simulink library "dkc"  (R2021b)
settings: Solver=VariableStepAuto  StartTime=0.0  StopTime=10.0  RelTol=1e-3
undefined symbols (not defined in the file or in its folder): ENUM_ANTITHEFT_ALARM, ENUM_ANTITHEFT_ARM, ENUM_ANTITHEFT_DISARM, ENUM_ANTITHEFT_WAIT, ENUM_BTCONNSTA_CONNECTED, ENUM_BTConnSta_CONNECTED, ENUM_BTCONNSTA_DISCONNECTED, ENUM_DKCAuthSta_DECRYPTIONFAIL, ENUM_DKCAuthSta_NORMAL, ENUM_DKCAuthSta_TIMEERROR, ENUM_DKCPCMDHANDING_FORCELIFT, ENUM_DKCPCMDHANDING_LOCK, ENUM_DKCPCMDHANDING_LOCKTGATEFAIL, ENUM_DKCPCMDHANDING_OVER, ENUM_DKCPCMDHANDING_TGATEHANDLE, ENUM_DKCPCMDHANDING_UNLOCK, ENUM_DkeyShowIVI_DEFAULT, ENUM_DkeyShowIVI_INVALID, ENUM_DkeyShowIVI_NFCGREEN, ENUM_DkeyShowIVI_NFCRED, ENUM_GEARACTUALPOSN_N, ENUM_GEARACTUALPOSN_P, ENUM_KEYMISSSTA_DEFAULT, ENUM_KEYMISSSTA_KEYMISS, ENUM_KEYMODE_DAFAULT, ENUM_KEYMODE_INVALID, ENUM_KEYMODE_NFC, ENUM_KEYMODE_UIDBLE, ENUM_KEYMODE_UIDUWB, ENUM_KEYTYPE_NFC, ENUM_KEYTYPE_NOREQ, ENUM_KEYTYPE_UID, ENUM_PCMDTOBCM_DEFAULT, ENUM_PCMDTOBCM_FORCELIFT, ENUM_PCMDTOBCM_LOCK, ENUM_PCMDTOBCM_LOCKTGATEFAIL, ENUM_PCMDTOBCM_NFCCOMMAND, ENUM_PCMDTOBCM_REMOTETGATE, ENUM_PCMDTOBCM_TGATEHANDLE, ENUM_PCMDTOBCM_UNLOCK, ENUM_PCMDTOBCM_UWBLOCK, ENUM_PCMDTOBCM_UWBUNLOCK, ENUM_PDKEYPTGRAW_INTOZONE, ENUM_PDKEYPTGRAW_OUTZONE, ENUM_PDKEYPTGRAW_UNAVALIABLE, ENUM_PDKEYRAWLULOCK_INLOCK, ENUM_PDKEYRAWLULOCK_INUNLOCK, ENUM_PDKEYRAWLULOCK_UNAVALIABLE, ENUM_PDKEYRAWPS_INPS, ENUM_PDKEYRAWPS_OUTPS, ENUM_PDKEYRAWPS_UNAVALIABLE, ENUM_PDKEYSPTGRAW_INTOZONE, ENUM_PDKEYSPTGRAW_OUTZONE, ENUM_PDKEYSPTGRAW_UNAVALIABLE, ENUM_PDKEYWELCOMERAW_INTOZONE, ENUM_PDKEYWELCOMERAW_UNAVALIABLE, ENUM_POWERSTA_OFF, ENUM_POWERSTA_OFFA, ENUM_POWERSTA_OFFC, ENUM_POWERSTA_ON ... (+79)
libraries: simulink x99, hcu_lib x6
(part 4 of 4)

== stateflow chart dkc/DKC/Subsystem/DKC_Handler/PTG_PCMD_Chart ==
  state PTG_CMDJudge
    state PrsSW1TailgateTimeoutLock_Cmd_Delay
      (default) -> (junction 154) : {
          |  VDKC_CmdDelayTime_s = 0;
          |  VDKC_CmdDelayDone_flg = FALSE;
          | }
      PrsSW1TailgateTimeoutLock_Cmd_Delay -> (junction 154) [order 1]
      (junction 154) -> (junction 155) [order 1] : [ VDKC_CmdDelayTime_s > KDKC_LockCmdDelayTime_s]
      (junction 154) -> (junction 156) [order 2]
      (junction 155) -> (junction 160) : {
          |  VDKC_CmdDelayDone_flg = TRUE;
          | }
      (junction 156) -> (junction 157) [order 1] : [ VDKC_PCmdFallingEdge_flg == TRUE]
      (junction 156) -> (junction 158) [order 2] : {
          |  VDKC_CmdDelayTime_s += task_time_s;
          | }
      (junction 157) -> (junction 159) : {
          |  VDKC_CmdDelayDone_flg = TRUE;
          | }
      (junction 159) -> (junction 158)
      (junction 160) -> (junction 159)
    state PrsSW2TailgateTimeoutLock_Cmd_Delay
      (default) -> (junction 225) : {
          |  VDKC_CmdDelayTime_s = 0;
          |  VDKC_CmdDelayDone_flg = FALSE;
          | }
      PrsSW2TailgateTimeoutLock_Cmd_Delay -> (junction 225) [order 1]
      (junction 225) -> (junction 226) [order 1] : [ VDKC_CmdDelayTime_s > KDKC_LockCmdDelayTime_s]
      (junction 225) -> (junction 227) [order 2]
      (junction 226) -> (junction 231) : {
          |  VDKC_CmdDelayDone_flg = TRUE;
          | }
      (junction 227) -> (junction 228) [order 1] : [ VDKC_PCmdFallingEdge_flg == TRUE]
      (junction 227) -> (junction 229) [order 2] : {
          |  VDKC_CmdDelayTime_s += task_time_s;
          | }
      (junction 228) -> (junction 230) : {
          |  VDKC_CmdDelayDone_flg = TRUE;
          | }
      (junction 230) -> (junction 229)
      (junction 231) -> (junction 230)
    state TailgateLockFail_Cmd_Delay
      (default) -> (junction 30) : {
          |  VDKC_CmdDelayTime_s = 0;
          |  VDKC_CmdDelayDone_flg = FALSE;
          | }
      TailgateLockFail_Cmd_Delay -> (junction 30) [order 1]
      (junction 30) -> (junction 35) [order 1] : [ VDKC_CmdDelayTime_s > KDKC_LockCmdDelayTime_s]
      (junction 30) -> (junction 33) [order 2]
      (junction 35) -> (junction 106) : {
          |  VDKC_CmdDelayDone_flg = TRUE;
          | }
      (junction 33) -> (junction 109) [order 1] : [ VDKC_PCmdFallingEdge_flg == TRUE]
      (junction 33) -> (junction 105) [order 2] : {
          |  VDKC_CmdDelayTime_s += task_time_s;
          | }
      (junction 109) -> (junction 107) : {
          |  VDKC_CmdDelayDone_flg = TRUE;
          | }
      (junction 107) -> (junction 105)
      (junction 106) -> (junction 107)
    state TailgateLock_Cmd_Delay
      (default) -> (junction 129) : {
          |  VDKC_CmdDelayTime_s = 0;
          |  VDKC_CmdDelayDone_flg = FALSE;
          | }
      TailgateLock_Cmd_Delay -> (junction 129) [order 1]
      (junction 129) -> (junction 130) [order 1] : [ VDKC_CmdDelayTime_s > KDKC_LockCmdDelayTime_s]
      (junction 129) -> (junction 131) [order 2]
      (junction 130) -> (junction 135) : {
          |  VDKC_CmdDelayDone_flg = TRUE;
          | }
      (junction 131) -> (junction 132) [order 1] : [ VDKC_PCmdFallingEdge_flg == TRUE]
      (junction 131) -> (junction 133) [order 2] : {
          |  VDKC_CmdDelayTime_s += task_time_s;
          | }
      (junction 132) -> (junction 134) : {
          |  VDKC_CmdDelayDone_flg = TRUE;
          | }
      (junction 134) -> (junction 133)
      (junction 135) -> (junction 134)
    state PTG_DKC_Cmd_Default
      en:
      VDKC_CmdHandling_flg = FALSE;
      VDKC_PTGPCmdToBCMRAW_enum = ENUM_PCMDTOBCM_DEFAULT;
      VDKC_PTGPCmdHandingSta_enum =ENUM_DKCPCMDHANDING_OVER;
    (default) -> (junction 8) : {VDKC_CmdHandling_flg = FALSE;}
    PTG_CMDJudge -> (junction 8) : [ !VDKC_CmdHandling_flg ]
    (junction 8) -> (junction 97) [order 1] : [ VDKC_PrsSW2TGFalEdgeOutPS_flg == TRUE&& VPMM_PowerSta_enum != ENUM_POWERSTA_READY]
    (junction 97) -> (junction 14) [order 1] : [ VBCM_AntitheftSta_enum ==ENUM_ANTITHEFT_DISARM ||...
        |   VBCM_AntitheftSta_enum == ENUM_ANTITHEFT_WAIT]
    (junction 8) -> (junction 84) [order 2]
    (junction 97) -> PTG_DKC_Cmd_Default [order 2]
    (junction 14) -> TailgateLock_Cmd_Delay : {
        | VDKC_CmdHandling_flg = TRUE;
        | VDKC_PTGPCmdToBCMRAW_enum = ENUM_PCMDTOBCM_LOCK;
        | VDKC_PTGPCmdHandingSta_enum =ENUM_DKCPCMDHANDING_LOCK;
        | }
    (junction 84) -> (junction 90) [order 1] : [ VDKC_PrsSW2TGFalEdgeInPS_flg == TRUE...
        | && VPMM_PowerSta_enum != ENUM_POWERSTA_READY
        | ]
    (junction 84) -> (junction 181) [order 2]
    (junction 90) -> (junction 211)
    (junction 181) -> (junction 183) [order 1] : [ VDKC_TGFalEdgeInPS_flg == TRUE...
        | &&VPMM_PowerSta_enum != ENUM_POWERSTA_READY
        | ]
    (junction 183) -> (junction 211) [order 1] : [ VBCM_AntitheftSta_enum ==ENUM_ANTITHEFT_ARM ||...
        |   VBCM_AntitheftSta_enum == ENUM_ANTITHEFT_ALARM]
    (junction 181) -> (junction 218) [order 2]
    (junction 183) -> PTG_DKC_Cmd_Default [order 2]
    (junction 211) -> TailgateLockFail_Cmd_Delay : {
        | VDKC_CmdHandling_flg = TRUE;
        | VDKC_PTGPCmdToBCMRAW_enum = ENUM_PCMDTOBCM_LOCKTGATEFAIL;
        | VDKC_PTGPCmdHandingSta_enum =ENUM_DKCPCMDHANDING_LOCKTGATEFAIL;
        | }
    (junction 218) -> (junction 220) [order 1] : [ VDKC_PrsSW2TGNoEdgeTimeOut_flg == TRUE]
        | %VPMM_PowerSta_enum != ENUM_POWERSTA_READY
        | %For reminding user that tailgate close fail when in READY
    (junction 218) -> (junction 148) [order 2]
    (junction 220) -> PrsSW2TailgateTimeoutLock_Cmd_Delay : {
        | VDKC_CmdHandling_flg = TRUE;
        | VDKC_PTGPCmdToBCMRAW_enum = ENUM_PCMDTOBCM_LOCK;
        | VDKC_PTGPCmdHandingSta_enum =ENUM_DKCPCMDHANDING_LOCK;
        | %VDKC_PTGPCmdToBCMRAW_enum =ENUM_PCMDTOBCM_CARSEARCHMUTE;
        | %VDKC_PTGPCmdHandingSta_enum =ENUM_DKCPCMDHANDING_CARSEARCH;
        | }
    (junction 148) -> (junction 150) [order 1] : [ VDKC_PrsSW1orDKCNoEdgTimOut_flg == TRUE]
        | %VPMM_PowerSta_enum != ENUM_POWERSTA_READY
        | %For reminding user that tailgate close fail when in READY
    (junction 150) -> (junction 250) [order 1] : [VBCM_AntitheftSta_enum ==ENUM_ANTITHEFT_ARM ||...
        |   VBCM_AntitheftSta_enum == ENUM_ANTITHEFT_ALARM]
    (junction 148) -> PTG_DKC_Cmd_Default [order 2]
    (junction 150) -> PTG_DKC_Cmd_Default [order 2]
    (junction 250) -> PrsSW1TailgateTimeoutLock_Cmd_Delay : {
        | VDKC_CmdHandling_flg = TRUE;
        | VDKC_PTGPCmdToBCMRAW_enum = ENUM_PCMDTOBCM_LOCK;
        | VDKC_PTGPCmdHandingSta_enum =ENUM_DKCPCMDHANDING_LOCK;
        | %VDKC_PTGPCmdToBCMRAW_enum =ENUM_PCMDTOBCM_CARSEARCHMUTE;
        | %VDKC_PTGPCmdHandingSta_enum =ENUM_DKCPCMDHANDING_CARSEARCH;
        | }
    PrsSW1TailgateTimeoutLock_Cmd_Delay -> PTG_DKC_Cmd_Default [order 1] : [ VDKC_CmdDelayDone_flg ]
    PrsSW2TailgateTimeoutLock_Cmd_Delay -> PTG_DKC_Cmd_Default [order 1] : [ VDKC_CmdDelayDone_flg ]
    TailgateLockFail_Cmd_Delay -> PTG_DKC_Cmd_Default [order 1] : [ VDKC_CmdDelayDone_flg ]
    TailgateLock_Cmd_Delay -> PTG_DKC_Cmd_Default [order 1] : [ VDKC_CmdDelayDone_flg ]
  data: KDKC_LockCmdDelayTime_s input single; VBCM_AntitheftSta_enum input uint8; VDKC_PrsSW2TGFalEdgeOutPS_flg input boolean; VDKC_PrsSW2TGFalEdgeInPS_flg input boolean; VDKC_TGFalEdgeInPS_flg input boolean; VDKC_PrsSW2TGNoEdgeTimeOut_flg input boolean; VDKC_PrsSW1orDKCNoEdgTimOut_flg input boolean; task_time_s input single; VPMM_PowerSta_enum input uint8; VDKC_CmdHandling_flg local boolean; VDKC_CmdDelayTime_s local single; ENUM_PCMDTOBCM_DEFAULT parameter; ENUM_PCMDTOBCM_LOCK parameter; FALSE parameter; TRUE parameter; ENUM_ANTITHEFT_DISARM parameter; ENUM_ANTITHEFT_WAIT parameter; ENUM_DKCPCMDHANDING_LOCK parameter; ENUM_DKCPCMDHANDING_OVER parameter; VDKC_PCmdFallingEdge_flg input boolean; VDKC_CmdDelayDone_flg local boolean; VDKC_PTGPCmdToBCMRAW_enum output uint8; VDKC_PTGPCmdHandingSta_enum output uint8; ENUM_DKCPCMDHANDING_LOCKTGATEFAIL parameter; ENUM_PCMDTOBCM_LOCKTGATEFAIL parameter; ENUM_POWERSTA_READY parameter; ENUM_ANTITHEFT_ALARM parameter; ENUM_ANTITHEFT_ARM parameter

== stateflow chart dkc/DKC/Subsystem/DKC_Handler/AllowSleep_Chart ==
  state FDCDKCAllowSleep
    (default) -> (junction 5) : {
        | VDKC_FDCKeyAllowSleep_flg=1;
        | VDKC_AllowSleepDelayTime_s=0;
        | }
    (junction 5) -> (junction 10) [order 1] : [VDKC_FDCDKCTimerActive_flg==1]
    FDCDKCAllowSleep -> (junction 5)
    (junction 10) -> (junction 143) : {
        | VDKC_FDCKeyAllowSleep_flg=0;
        | VDKC_AllowSleepDelayTime_s=0;
        | }
    (junction 5) -> (junction 131) [order 2]
    (junction 131) -> (junction 133) [order 1] : [VPMM_PowerSta_enum==ENUM_POWERSTA_OFF]
    (junction 131) -> (junction 139) [order 2] : {
        | VDKC_FDCKeyAllowSleep_flg=0;
        | VDKC_AllowSleepDelayTime_s=0;
        | }
    (junction 133) -> (junction 135)
    (junction 135) -> (junction 147) [order 1] : [VDKC_AllowSleepDelayTime_s>KDKC_DKCAllowSleepDelayTime_s]
    (junction 135) -> (junction 151) [order 2] : {
        | VDKC_AllowSleepDelayTime_s+=task_time_s;
        | }
    (junction 147) -> (junction 149) : {
        | VDKC_FDCKeyAllowSleep_flg=1;
        | }
    (junction 151) -> (junction 139)
    (junction 149) -> (junction 151)
    (junction 143) -> (junction 149)
  data: KDKC_DKCAllowSleepDelayTime_s input single; VDKC_FDCDKCTimerActive_flg input boolean; task_time_s input single; VPMM_PowerSta_enum input uint8; ENUM_POWERSTA_OFF parameter; VDKC_AllowSleepDelayTime_s local single; VDKC_FDCKeyAllowSleep_flg output boolean

== stateflow chart dkc/DKC/Subsystem/DKC_Handler/BTRSSIJudgeArea_Chart ==
  state BTRSSIJudgeArea_Chart
    (default) -> (junction 119) : {
        |  VDKC_RSSIJudgeArea_enum=ENUM_RSSIAREA_DAFAULT ;
        |  VDKC_RSSIConnCheckMode=0;%RSSIJudgeUnlockArea
        |  RSSIConnStrongDet_Cnt=0;
        |  RSSIConnWeakDet_Cnt=0;
        | }
    BTRSSIJudgeArea_Chart -> (junction 119)
    (junction 119) -> (junction 121) [order 1] : [VDKC_BTConnectSta_enum==ENUM_BTCONNSTA_CONNECTED]
    (junction 119) -> (junction 127) [order 2] : {
        |  VDKC_RSSIJudgeArea_enum=ENUM_RSSIAREA_DAFAULT ;%Output signal
        |  VDKC_RSSIConnCheckMode=0;%RSSIJudge Weak (Unlock) Area
        |  RSSIConnStrongDet_Cnt=0;
        |  RSSIConnWeakDet_Cnt=0;
        | }
    (junction 121) -> (junction 4) : {
        |
        | SampTimeCounter = SampTimeCounter + 1;
        | }
    (junction 4) -> (junction 9) [order 1] : [SampTimeCounter>=(KDKC_BTRSSISampTime_s/task_time_s)]
    (junction 4) -> (junction 11) [order 2]
    (junction 9) -> (junction 65) : {
        | SampTimeCounter=0;%add uwb area
        | }
    (junction 65) -> (junction 67) [order 1] : [VDKC_RSSIConnCheckMode==1]%RSSIJudgeLockArea_loop
    (junction 65) -> (junction 91) [order 2] : %RSSIJudgeUnlockArea_loop
    (junction 67) -> (junction 13)
    (junction 91) -> (junction 89) [order 1] : [VDKC_KeyUWBDetArea_enum==ENUM_UWBDET_PSZONE ||....
        | VDKC_KeyUWBDetArea_enum==ENUM_UWBDET_UNLOCKZONE ]
    (junction 13) -> (junction 170) [order 1] : [VDKC_KeyUWBDetArea_enum!=ENUM_UWBDET_PSZONE &&....
        | VDKC_KeyUWBDetArea_enum!=ENUM_UWBDET_UNLOCKZONE ]
    (junction 91) -> (junction 111) [order 2] : {
        | RSSIConnStrongDet_Cnt=0;
        | }
    (junction 89) -> (junction 93)
    (junction 13) -> (junction 106) [order 2] : {
        | RSSIConnWeakDet_Cnt=0;
        | }
    (junction 170) -> (junction 172)
    (junction 172) -> (junction 23) [order 1] : [  (VDKC_DKCBTRSSI_dB<=KDKC_JudBTRSSIWeakThres_dB&&VDKC_DKCBTRSSI_dB>=-100)||....
        |    (VDKC_DKCBTRSSI_dB==127)&&(VDKC_KeyUWBDetArea_enum==ENUM_UWBDET_UNAVALIABLE)    ]
        | %dB MIN=-100 (Valid Range:0~-100)
    (junction 93) -> (junction 84) [order 1] : [(VDKC_DKCBTRSSI_dB>=KDKC_JudBTRSSIStrongThres_dB&&VDKC_DKCBTRSSI_dB<=0)]
        | %dB MAX==0 (Valid Range:0~-100)
    (junction 172) -> (junction 174) [order 2] : {
        | RSSIConnWeakDet_Cnt=0;
        | }
    (junction 23) -> (junction 31) : {
        | RSSIConnWeakDet_Cnt++;
        | }
    (junction 93) -> (junction 109) [order 2] : {
        | RSSIConnStrongDet_Cnt=0;
        | }
    (junction 84) -> (junction 81) : {
        | RSSIConnStrongDet_Cnt++;
        | }
    (junction 81) -> (junction 144) [order 1] : [RSSIConnStrongDet_Cnt>KDKC_JudBTRSSIStrongDeb_cnt]
    (junction 81) -> (junction 148) [order 2]
    (junction 144) -> (junction 146) : {
        | VDKC_RSSIJudgeArea_enum=ENUM_RSSIAreaSta_STRONG;%Output signal
        | RSSIConnStrongDet_Cnt=0;
        | VDKC_RSSIConnCheckMode=1;%to RSSIJudge Weak Area loop
        | }
    (junction 31) -> (junction 156) [order 1] : [RSSIConnWeakDet_Cnt>KDKC_JudBTRSSIWeakDeb_cnt]
    (junction 31) -> (junction 104) [order 2]
    (junction 156) -> (junction 159) : {
        | VDKC_RSSIJudgeArea_enum=ENUM_RSSIAREA_WEAK;%Output signal
        | RSSIConnWeakDet_Cnt=0;
        | VDKC_RSSIConnCheckMode=0;%to RSSIJudge strong Area loop
        | }
    (junction 11) -> (junction 127)
    (junction 111) -> (junction 11)
    (junction 109) -> (junction 111)
    (junction 148) -> (junction 109)
    (junction 146) -> (junction 148)
    (junction 106) -> (junction 146)
    (junction 174) -> (junction 106)
    (junction 104) -> (junction 174)
    (junction 159) -> (junction 104)
  data: VDKC_DKCBTRSSI_dB input; KDKC_JudBTRSSIWeakThres_dB input; KDKC_JudBTRSSIStrongThres_dB input; KDKC_JudBTRSSIWeakDeb_cnt input; KDKC_JudBTRSSIStrongDeb_cnt input; KDKC_BTRSSISampTime_s input; VDKC_BTConnectSta_enum input; VDKC_KeyUWBDetArea_enum input; task_time_s input; SampTimeCounter local single; ENUM_BTCONNSTA_CONNECTED parameter; ENUM_UWBDET_UNLOCKZONE parameter; ENUM_UWBDET_PSZONE parameter; ENUM_RSSIAreaSta_STRONG parameter; ENUM_RSSIAREA_DAFAULT parameter; ENUM_RSSIAREA_WEAK parameter; VDKC_RSSIJudgeArea_enum output uint8; VDKC_RSSIConnCheckMode local uint8; RSSIConnWeakDet_Cnt local uint16; RSSIConnStrongDet_Cnt local uint16; ENUM_UWBDET_UNAVALIABLE parameter

== stateflow chart dkc/DKC/Subsystem/DKC_Handler/AutoLock_PCMD_Chart ==
  state AutoLock
    state AutoLock_Cmd_Delay
      (default) -> (junction 30) : {
          |  VDKC_CmdDelayTime_s = 0;
          |  VDKC_CmdDelayDone_flg = FALSE;
          | }
      AutoLock_Cmd_Delay -> (junction 30) [order 1]
      (junction 30) -> (junction 35) [order 1] : [ VDKC_CmdDelayTime_s > KDKC_LockCmdDelayTime_s]
      (junction 30) -> (junction 33) [order 2]
      (junction 35) -> (junction 106) : {
          |  VDKC_CmdDelayDone_flg = TRUE;
          | }
      (junction 33) -> (junction 109) [order 1] : [ VDKC_PCmdFallingEdge_flg == TRUE]
      (junction 33) -> (junction 105) [order 2] : {
          |  VDKC_CmdDelayTime_s += task_time_s;
          | }
      (junction 109) -> (junction 107) : {
          |  VDKC_CmdDelayDone_flg = TRUE;
          | }
      (junction 107) -> (junction 105)
      (junction 106) -> (junction 107)
    state AutoFORCELIFT_Cmd_Delay
      (default) -> (junction 136) : {
          |  VDKC_CmdDelayTime_s = 0;
          |  VDKC_CmdDelayDone_flg = FALSE;
          | }
      AutoFORCELIFT_Cmd_Delay -> (junction 136) [order 1]
      (junction 136) -> (junction 137) [order 1] : [ VDKC_CmdDelayTime_s > KDKC_LockCmdDelayTime_s]
      (junction 136) -> (junction 138) [order 2]
      (junction 137) -> (junction 142) : {
          |  VDKC_CmdDelayDone_flg = TRUE;
          | }
      (junction 138) -> (junction 139) [order 1] : [ VDKC_PCmdFallingEdge_flg == TRUE]
      (junction 138) -> (junction 140) [order 2] : {
          |  VDKC_CmdDelayTime_s += task_time_s;
          | }
      (junction 139) -> (junction 141) : {
          |  VDKC_CmdDelayDone_flg = TRUE;
          | }
      (junction 141) -> (junction 140)
      (junction 142) -> (junction 141)
    state AutoLock_DKC_Cmd_Default
      en:
      VDKC_CmdHandling_flg = FALSE;
      VDKC_AutoLockPCmdToBCMRAW_enum = ENUM_PCMDTOBCM_DEFAULT;
      VDKC_AutoLockPCmdHandingSta_enum=ENUM_DKCPCMDHANDING_OVER;
    (default) -> (junction 5) : {VDKC_CmdHandling_flg = FALSE;}
    AutoLock -> (junction 5) : [ !VDKC_CmdHandling_flg ]
    (junction 5) -> (junction 10) [order 1] : [ VPMM_PowerSta_enum == ENUM_POWERSTA_READY&&VDKC_PMMChgToReady_flg==TRUE]
    (junction 5) -> (junction 84) [order 2]
    (junction 10) -> (junction 131)
    (junction 131) -> (junction 133) [order 1] : [ VBCM_AntitheftSta_enum ==ENUM_ANTITHEFT_ARM ||...
        |   VBCM_AntitheftSta_enum == ENUM_ANTITHEFT_ALARM]
    (junction 84) -> (junction 87) [order 1] : [ VPMM_PowerSta_enum != ENUM_POWERSTA_READY&&VDKC_AutoLockReqtoLock_flg == TRUE]
    (junction 131) -> AutoLock_DKC_Cmd_Default [order 2]
    (junction 133) -> AutoFORCELIFT_Cmd_Delay : {
        | VDKC_CmdHandling_flg = TRUE;
        | VDKC_AutoLockPCmdToBCMRAW_enum = ENUM_PCMDTOBCM_FORCELIFT;
        | VDKC_AutoLockPCmdHandingSta_enum =ENUM_DKCPCMDHANDING_FORCELIFT;
        | }
    (junction 84) -> AutoLock_DKC_Cmd_Default [order 2]
    (junction 87) -> (junction 91)
    (junction 91) -> (junction 90) [order 1] : [ VBCM_AntitheftSta_enum ==ENUM_ANTITHEFT_DISARM ||...
        |   VBCM_AntitheftSta_enum == ENUM_ANTITHEFT_WAIT]
    (junction 91) -> AutoLock_DKC_Cmd_Default [order 2]
    (junction 90) -> AutoLock_Cmd_Delay : {
        | VDKC_CmdHandling_flg = TRUE;
        | VDKC_AutoLockPCmdToBCMRAW_enum = ENUM_PCMDTOBCM_LOCK;
        | VDKC_AutoLockPCmdHandingSta_enum =ENUM_DKCPCMDHANDING_LOCK;
        | }
    AutoLock_Cmd_Delay -> AutoLock_DKC_Cmd_Default [order 1] : [ VDKC_CmdDelayDone_flg ]
    AutoFORCELIFT_Cmd_Delay -> AutoLock_DKC_Cmd_Default [order 1] : [ VDKC_CmdDelayDone_flg ]
  data: KDKC_LockCmdDelayTime_s input single; VBCM_AntitheftSta_enum input uint8; VDKC_AutoLockReqtoLock_flg input boolean; VDKC_PMMChgToReady_flg input boolean; task_time_s input single; VDKC_CmdHandling_flg local boolean; VDKC_CmdDelayTime_s local single; ENUM_PCMDTOBCM_DEFAULT parameter; ENUM_PCMDTOBCM_LOCK parameter; FALSE parameter; TRUE parameter; ENUM_POWERSTA_READY parameter; VPMM_PowerSta_enum input uint8; ENUM_ANTITHEFT_DISARM parameter; ENUM_ANTITHEFT_WAIT parameter; ENUM_DKCPCMDHANDING_LOCK parameter; ENUM_DKCPCMDHANDING_OVER parameter; VDKC_PCmdFallingEdge_flg input boolean; VDKC_AutoLockPCmdToBCMRAW_enum output uint8; VDKC_AutoLockPCmdHandingSta_enum output uint8; VDKC_CmdDelayDone_flg local boolean; ENUM_ANTITHEFT_ARM parameter; ENUM_ANTITHEFT_ALARM parameter; ENUM_DKCPCMDHANDING_FORCELIFT parameter; ENUM_PCMDTOBCM_FORCELIFT parameter

== stateflow chart dkc/DKC/Subsystem/DKC_Handler/NFC_PCMD_Chart ==
  state NFC
    state NFCLock_Cmd_Delay
      (default) -> (junction 30) : {
          |  VDKC_CmdDelayTime_s = 0;
          |  VDKC_CmdDelayDone_flg = FALSE;
          | }
      NFCLock_Cmd_Delay -> (junction 30) [order 1]
      (junction 30) -> (junction 35) [order 1] : [ VDKC_CmdDelayTime_s > KDKC_LockCmdDelayTime_s]
      (junction 30) -> (junction 86) [order 2]
      (junction 35) -> (junction 37) : {
          |  VDKC_CmdDelayDone_flg = TRUE;
          | }
      (junction 86) -> (junction 88) [order 1] : [ VDKC_PCmdFallingEdge_flg == TRUE]
      (junction 88) -> (junction 94) : {
          |  VDKC_CmdDelayDone_flg = TRUE;
          | }
      (junction 86) -> (junction 33) [order 2] : {
          |  VDKC_CmdDelayTime_s += task_time_s;
          | }
      (junction 94) -> (junction 33)
      (junction 37) -> (junction 94)
    state NFCUnlock_Cmd_Delay
      (default) -> (junction 47) : {
          |  VDKC_CmdDelayTime_s = 0;
          |  VDKC_CmdDelayDone_flg = FALSE;
          | }
      NFCUnlock_Cmd_Delay -> (junction 47) [order 1]
      (junction 47) -> (junction 45) [order 1] : [ VDKC_CmdDelayTime_s > KDKC_UnlockCmdDelayTime_s]
      (junction 47) -> (junction 97) [order 2]
      (junction 45) -> (junction 49) : {
          |  VDKC_CmdDelayDone_flg = TRUE;
          | }
      (junction 97) -> (junction 99) [order 1] : [ VDKC_PCmdFallingEdge_flg == TRUE]
      (junction 97) -> (junction 53) [order 2] : {
          |  VDKC_CmdDelayTime_s += task_time_s;
          | }
      (junction 99) -> (junction 101) : {
          |  VDKC_CmdDelayDone_flg = TRUE;
          | }
      (junction 49) -> (junction 101)
      (junction 101) -> (junction 53)
    state NFC_DKC_Cmd_Default
      en:
      VDKC_CmdHandling_flg = FALSE;
      VDKC_NFCPCmdToBCMRAW_enum = ENUM_PCMDTOBCM_DEFAULT;
      VDKC_NFCPCmdHandingSta_enum=ENUM_DKCPCMDHANDING_OVER ;
    (default) -> (junction 5) : {VDKC_CmdHandling_flg = FALSE;}
    NFC -> (junction 5) : [ !VDKC_CmdHandling_flg ]
    (junction 5) -> (junction 10) [order 2]
    (junction 5) -> (junction 8) [order 1] : [ VDKC_DetectNFCRisingEdge_flg  && VPMM_PowerSta_enum != ENUM_POWERSTA_READY]
    (junction 10) -> NFC_DKC_Cmd_Default
    (junction 8) -> (junction 14) [order 1] : [ VBCM_AntitheftSta_enum == ENUM_ANTITHEFT_ARM ||...
        |   VBCM_AntitheftSta_enum == ENUM_ANTITHEFT_ALARM ]
    (junction 8) -> NFCLock_Cmd_Delay [order 2] : %AntitheftSta == DISARM or WAIT
        |
        | { VDKC_CmdHandling_flg = TRUE;
        |   VDKC_NFCPCmdToBCMRAW_enum = ENUM_PCMDTOBCM_LOCK ;
        |   VDKC_NFCPCmdHandingSta_enum=ENUM_DKCPCMDHANDING_LOCK;
        | }
    (junction 14) -> NFCUnlock_Cmd_Delay : { VDKC_CmdHandling_flg = TRUE;
        |   VDKC_NFCPCmdToBCMRAW_enum =ENUM_PCMDTOBCM_UNLOCK;
        |   VDKC_NFCPCmdHandingSta_enum=ENUM_DKCPCMDHANDING_UNLOCK;
        | }
    NFCLock_Cmd_Delay -> NFC_DKC_Cmd_Default [order 1] : [ VDKC_CmdDelayDone_flg ]
    NFCUnlock_Cmd_Delay -> NFC_DKC_Cmd_Default [order 1] : [ VDKC_CmdDelayDone_flg ]
  data: KDKC_LockCmdDelayTime_s input single; KDKC_UnlockCmdDelayTime_s input single; VBCM_AntitheftSta_enum input uint8; VDKC_DetectNFCRisingEdge_flg input boolean; task_time_s input single; VDKC_CmdHandling_flg local boolean; VDKC_CmdDelayTime_s local single; ENUM_ANTITHEFT_ALARM parameter; ENUM_ANTITHEFT_ARM parameter; ENUM_PCMDTOBCM_DEFAULT parameter; FALSE parameter; TRUE parameter; VDKC_NFCPCmdToBCMRAW_enum output uint8; ENUM_POWERSTA_READY parameter; VPMM_PowerSta_enum input uint8; VDKC_NFCPCmdHandingSta_enum output uint8; ENUM_DKCPCMDHANDING_LOCK parameter; ENUM_DKCPCMDHANDING_UNLOCK parameter; ENUM_DKCPCMDHANDING_OVER parameter; VDKC_PCmdFallingEdge_flg input boolean; VDKC_CmdDelayDone_flg local boolean; ENUM_PCMDTOBCM_UNLOCK parameter; ENUM_PCMDTOBCM_LOCK parameter

== stateflow chart dkc/DKC/Subsystem/DKC_Handler/UIDButton_PCMD_Chart ==
  state BLEButton
    state UIDButtonUnlock_Cmd_Delay
      (default) -> (junction 47) : {
          |  VDKC_CmdDelayTime_s = 0;
          |  VDKC_CmdDelayDone_flg = FALSE;
          | }
      UIDButtonUnlock_Cmd_Delay -> (junction 47) [order 1]
      (junction 47) -> (junction 45) [order 1] : [ VDKC_CmdDelayTime_s > KDKC_UnlockCmdDelayTime_s]
      (junction 47) -> (junction 53) [order 2]
      (junction 45) -> (junction 117) : {
          |  VDKC_CmdDelayDone_flg = TRUE;
          | }
      (junction 53) -> (junction 118) [order 1] : [ VDKC_PCmdFallingEdge_flg == TRUE]
      (junction 53) -> (junction 115) [order 2] : {
          |  VDKC_CmdDelayTime_s += task_time_s;
          | }
      (junction 118) -> (junction 116) : {
          |  VDKC_CmdDelayDone_flg = TRUE;
          | }
      (junction 116) -> (junction 115)
      (junction 117) -> (junction 116)
    state UIDButtonLock_Cmd_Delay
      (default) -> (junction 30) : {
          |  VDKC_CmdDelayTime_s = 0;
          |  VDKC_CmdDelayDone_flg = FALSE;
          | }
      UIDButtonLock_Cmd_Delay -> (junction 30) [order 1]
      (junction 30) -> (junction 35) [order 1] : [ VDKC_CmdDelayTime_s > KDKC_LockCmdDelayTime_s]
      (junction 30) -> (junction 33) [order 2]
      (junction 35) -> (junction 106) : {
          |  VDKC_CmdDelayDone_flg = TRUE;
          | }
      (junction 33) -> (junction 109) [order 1] : [ VDKC_PCmdFallingEdge_flg == TRUE]
      (junction 33) -> (junction 105) [order 2] : {
          |  VDKC_CmdDelayTime_s += task_time_s;
          | }
      (junction 109) -> (junction 107) : {
          |  VDKC_CmdDelayDone_flg = TRUE;
          | }
      (junction 107) -> (junction 105)
      (junction 106) -> (junction 107)
    state UIDButtonReTailGate_Cmd_Delay
      (default) -> (junction 167) : {
          |  VDKC_CmdDelayTime_s = 0;
          |  VDKC_CmdDelayDone_flg = FALSE;
          | }
      UIDButtonReTailGate_Cmd_Delay -> (junction 167) [order 1]
      (junction 167) -> (junction 168) [order 1] : [ VDKC_CmdDelayTime_s > KDKC_LockCmdDelayTime_s]
      (junction 167) -> (junction 169) [order 2]
      (junction 168) -> (junction 173) : {
          |  VDKC_CmdDelayDone_flg = TRUE;
          | }
      (junction 169) -> (junction 170) [order 1] : [ VDKC_PCmdFallingEdge_flg == TRUE]
      (junction 170) -> (junction 172) : {
          |  VDKC_CmdDelayDone_flg = TRUE;
          | }
      (junction 169) -> (junction 171) [order 2] : {
          |  VDKC_CmdDelayTime_s += task_time_s;
          | }
      (junction 172) -> (junction 171)
      (junction 173) -> (junction 172)
    state UIDButtonChargeCover_Cmd_Delay
      (default) -> (junction 303) : {
          |  VDKC_CmdDelayTime_s = 0;
          |  VDKC_CmdDelayDone_flg = FALSE;
          | }
      UIDButtonChargeCover_Cmd_Delay -> (junction 303) [order 1]
      (junction 303) -> (junction 304) [order 1] : [ VDKC_CmdDelayTime_s > KDKC_LockCmdDelayTime_s]
      (junction 303) -> (junction 305) [order 2]
      (junction 304) -> (junction 309) : {
          |  VDKC_CmdDelayDone_flg = TRUE;
          | }
      (junction 305) -> (junction 306) [order 1] : [ VDKC_PCmdFallingEdge_flg == TRUE]
      (junction 305) -> (junction 307) [order 2] : {
          |  VDKC_CmdDelayTime_s += task_time_s;
          | }
      (junction 306) -> (junction 308) : {
          |  VDKC_CmdDelayDone_flg = TRUE;
          | }
      (junction 308) -> (junction 307)
      (junction 309) -> (junction 308)
    state UIDButtonFrontHood_Cmd_Delay
      (default) -> (junction 264) : {
          |  VDKC_CmdDelayTime_s = 0;
          |  VDKC_CmdDelayDone_flg = FALSE;
          | }
      UIDButtonFrontHood_Cmd_Delay -> (junction 264) [order 1]
      (junction 264) -> (junction 265) [order 1] : [ VDKC_CmdDelayTime_s > KDKC_LockCmdDelayTime_s]
      (junction 264) -> (junction 266) [order 2]
      (junction 265) -> (junction 270) : {
          |  VDKC_CmdDelayDone_flg = TRUE;
          | }
      (junction 266) -> (junction 267) [order 1] : [ VDKC_PCmdFallingEdge_flg == TRUE]
      (junction 266) -> (junction 268) [order 2] : {
          |  VDKC_CmdDelayTime_s += task_time_s;
          | }
      (junction 267) -> (junction 269) : {
          |  VDKC_CmdDelayDone_flg = TRUE;
          | }
      (junction 269) -> (junction 268)
      (junction 270) -> (junction 269)
    state UIDButtonCarSearch_Cmd_Delay
      (default) -> (junction 198) : {
          |  VDKC_CmdDelayTime_s = 0;
          |  VDKC_CmdDelayDone_flg = FALSE;
          | }
      UIDButtonCarSearch_Cmd_Delay -> (junction 198) [order 1]
      (junction 198) -> (junction 199) [order 1] : [ VDKC_CmdDelayTime_s > KDKC_LockCmdDelayTime_s]
      (junction 198) -> (junction 200) [order 2]
      (junction 199) -> (junction 204) : {
          |  VDKC_CmdDelayDone_flg = TRUE;
          | }
      (junction 200) -> (junction 201) [order 1] : [ VDKC_PCmdFallingEdge_flg == TRUE]
      (junction 200) -> (junction 202) [order 2] : {
          |  VDKC_CmdDelayTime_s += task_time_s;
          | }
      (junction 201) -> (junction 203) : {
          |  VDKC_CmdDelayDone_flg = TRUE;
          | }
      (junction 203) -> (junction 202)
      (junction 204) -> (junction 203)
    state UIDButton_DKC_Cmd_Default
      en:
      VDKC_CmdHandling_flg = FALSE;
      VDKC_UIDButtonPCmdToBCMRAW_enum = ENUM_PCMDTOBCM_DEFAULT;
      VDKC_UIDButtonPCmdHandingSta_enum=ENUM_DKCPCMDHANDING_OVER;
    (default) -> (junction 5) : {VDKC_CmdHandling_flg = FALSE;}
    (junction 5) -> (junction 14) [order 1] : [ VDKC_UIDButtonUnlock_flg == TRUE && VPMM_PowerSta_enum != ENUM_POWERSTA_READY]
    BLEButton -> (junction 5) : [ !VDKC_CmdHandling_flg ]
    (junction 14) -> UIDButtonUnlock_Cmd_Delay : {
        | VDKC_CmdHandling_flg = TRUE;
        | VDKC_UIDButtonPCmdToBCMRAW_enum = ENUM_PCMDTOBCM_UNLOCK;
        | VDKC_UIDButtonPCmdHandingSta_enum =ENUM_DKCPCMDHANDING_UNLOCK;
        | }
    (junction 5) -> (junction 134) [order 2]
    (junction 134) -> (junction 136) [order 1] : [ VDKC_UIDButtonLock_flg == TRUE && VPMM_PowerSta_enum != ENUM_POWERSTA_READY]
    (junction 136) -> UIDButtonLock_Cmd_Delay : {
        | VDKC_CmdHandling_flg = TRUE;
        | VDKC_UIDButtonPCmdToBCMRAW_enum = ENUM_PCMDTOBCM_LOCK;
        | VDKC_UIDButtonPCmdHandingSta_enum =ENUM_DKCPCMDHANDING_LOCK;
        | }
    (junction 134) -> (junction 138) [order 2]
    (junction 138) -> (junction 140) [order 1] : [VDKC_UIDButtonRemTailGate_flg==TRUE]
    (junction 140) -> (junction 150)
    (junction 138) -> (junction 142) [order 2]
    (junction 150) -> (junction 153) [order 1] : [VDKC_VehSpeed_kph<=0&&....
        |   (VDKC_GearActualPosn_enum==ENUM_GEARACTUALPOSN_P||....
        |    VDKC_GearActualPosn_enum==ENUM_GEARACTUALPOSN_N)]
    (junction 142) -> (junction 144) [order 1] : [VDKC_UIDButtonCarSearch_flg==TRUE]
    (junction 144) -> (junction 217)
    (junction 150) -> UIDButton_DKC_Cmd_Default [order 2]
    (junction 153) -> UIDButtonReTailGate_Cmd_Delay : {
        | VDKC_CmdHandling_flg = TRUE;
        | VDKC_UIDButtonPCmdToBCMRAW_enum =ENUM_PCMDTOBCM_REMOTETGATE ;
        | VDKC_UIDButtonPCmdHandingSta_enum =ENUM_DKCPCMDHANDING_REMTAILGATE ;
        | }
    (junction 142) -> (junction 231) [order 2]
    UIDButtonUnlock_Cmd_Delay -> UIDButton_DKC_Cmd_Default [order 1] : [ VDKC_CmdDelayDone_flg ]
    (junction 231) -> (junction 281) [order 1] : [VDKC_UIDButtonFrontHood_flg==TRUE]
    (junction 281) -> (junction 282) [order 1] : [VDKC_VehSpeed_kph<=0&&....
        |   (VDKC_GearActualPosn_enum==ENUM_GEARACTUALPOSN_P||....
        |    VDKC_GearActualPosn_enum==ENUM_GEARACTUALPOSN_N)]
    (junction 217) -> (junction 219) [order 1] : [VDKC_VehSpeed_kph<=0]
    (junction 231) -> (junction 296) [order 2]
    (junction 281) -> UIDButton_DKC_Cmd_Default [order 2]
    (junction 282) -> UIDButtonFrontHood_Cmd_Delay : {
        | VDKC_CmdHandling_flg = TRUE;
        | VDKC_UIDButtonPCmdToBCMRAW_enum =ENUM_PCMDTOBCM_FRONTHOOD;
        | VDKC_UIDButtonPCmdHandingSta_enum =ENUM_DKCPCMDHANDING_FRONTHOOD;
        | }
    (junction 217) -> (junction 196) [order 2]
    (junction 219) -> (junction 192)
    UIDButtonLock_Cmd_Delay -> UIDButton_DKC_Cmd_Default [order 1] : [ VDKC_CmdDelayDone_flg ]
    (junction 296) -> (junction 298) [order 1] : [VDKC_UIDButtonChargeCover_flg==TRUE&& VPMM_PowerSta_enum != ENUM_POWERSTA_READY]
    (junction 296) -> UIDButton_DKC_Cmd_Default [order 2]
    (junction 298) -> UIDButtonChargeCover_Cmd_Delay : {
        | VDKC_CmdHandling_flg = TRUE;
        | VDKC_UIDButtonPCmdToBCMRAW_enum =ENUM_PCMDTOBCM_CHARGECOVER ;
        | VDKC_UIDButtonPCmdHandingSta_enum =ENUM_DKCPCMDHANDING_CHARGECOVER  ;
        | }
    (junction 196) -> (junction 192) [order 1] : [ VDKC_VehSpeed_kph>=0xFFF&&....
        |   (VDKC_GearActualPosn_enum==ENUM_GEARACTUALPOSN_P||....
        |    VDKC_GearActualPosn_enum==ENUM_GEARACTUALPOSN_N)]
    (junction 196) -> UIDButton_DKC_Cmd_Default [order 2]
    (junction 192) -> UIDButtonCarSearch_Cmd_Delay : {
        | VDKC_CmdHandling_flg = TRUE;
        | VDKC_UIDButtonPCmdToBCMRAW_enum =ENUM_PCMDTOBCM_CARSEARCH;
        | VDKC_UIDButtonPCmdHandingSta_enum =ENUM_DKCPCMDHANDING_CARSEARCH;
        | }
    UIDButtonReTailGate_Cmd_Delay -> UIDButton_DKC_Cmd_Default [order 1] : [ VDKC_CmdDelayDone_flg ]
    UIDButtonChargeCover_Cmd_Delay -> UIDButton_DKC_Cmd_Default [order 1] : [ VDKC_CmdDelayDone_flg ]
    UIDButtonFrontHood_Cmd_Delay -> UIDButton_DKC_Cmd_Default [order 1] : [ VDKC_CmdDelayDone_flg ]
    UIDButtonCarSearch_Cmd_Delay -> UIDButton_DKC_Cmd_Default [order 1] : [ VDKC_CmdDelayDone_flg ]
  data: KDKC_LockCmdDelayTime_s input single; KDKC_UnlockCmdDelayTime_s input single; VDKC_UIDButtonUnlock_flg input boolean; VDKC_UIDButtonLock_flg input boolean; VDKC_UIDButtonFrontHood_flg input boolean; VDKC_UIDButtonRemTailGate_flg input boolean; VDKC_UIDButtonChargeCover_flg input boolean; VDKC_UIDButtonCarSearch_flg input boolean; task_time_s input single; VDKC_CmdHandling_flg local boolean; VDKC_CmdDelayTime_s local single; ENUM_PCMDTOBCM_DEFAULT parameter; ENUM_PCMDTOBCM_LOCK parameter; ENUM_PCMDTOBCM_UNLOCK parameter; FALSE parameter; TRUE parameter; ENUM_POWERSTA_READY parameter; VPMM_PowerSta_enum input uint8; ENUM_DKCPCMDHANDING_LOCK parameter; ENUM_DKCPCMDHANDING_UNLOCK parameter; ENUM_DKCPCMDHANDING_OVER parameter; VDKC_UIDButtonPCmdToBCMRAW_enum output uint8; VDKC_UIDButtonPCmdHandingSta_enum output uint8; VDKC_VehSpeed_kph input; VDKC_GearActualPosn_enum input uint8; VDKC_PCmdFallingEdge_flg input boolean; ENUM_DKCPCMDHANDING_CARSEARCH parameter; ENUM_PCMDTOBCM_REMOTETGATE parameter; ENUM_DKCPCMDHANDING_REMTAILGATE parameter; ENUM_GEARACTUALPOSN_N parameter; ENUM_GEARACTUALPOSN_P parameter; ENUM_PCMDTOBCM_CARSEARCH parameter; ENUM_DKCPCMDHANDING_FRONTHOOD parameter; ENUM_PCMDTOBCM_CHARGECOVER parameter; ENUM_PCMDTOBCM_FRONTHOOD parameter; ENUM_DKCPCMDHANDING_CHARGECOVER parameter; VDKC_CmdDelayDone_flg local boolean
